simulink library "robot2"
libraries: AtomicLibrary x3, BusImpl x1

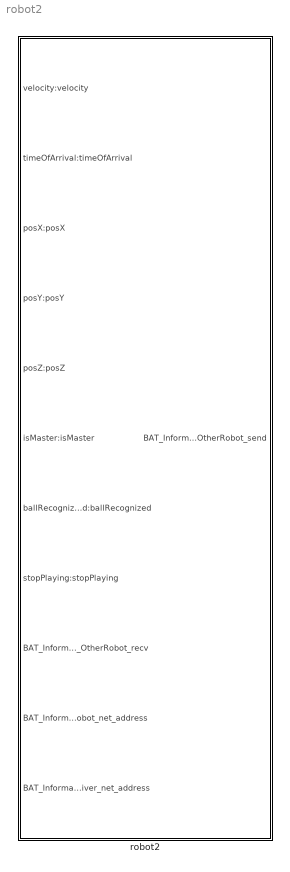
== system robot2 ==
  robot2 : Subsystem  Tag=id=_Sbbd0KYDEeKR7Lwk7UC7tQ

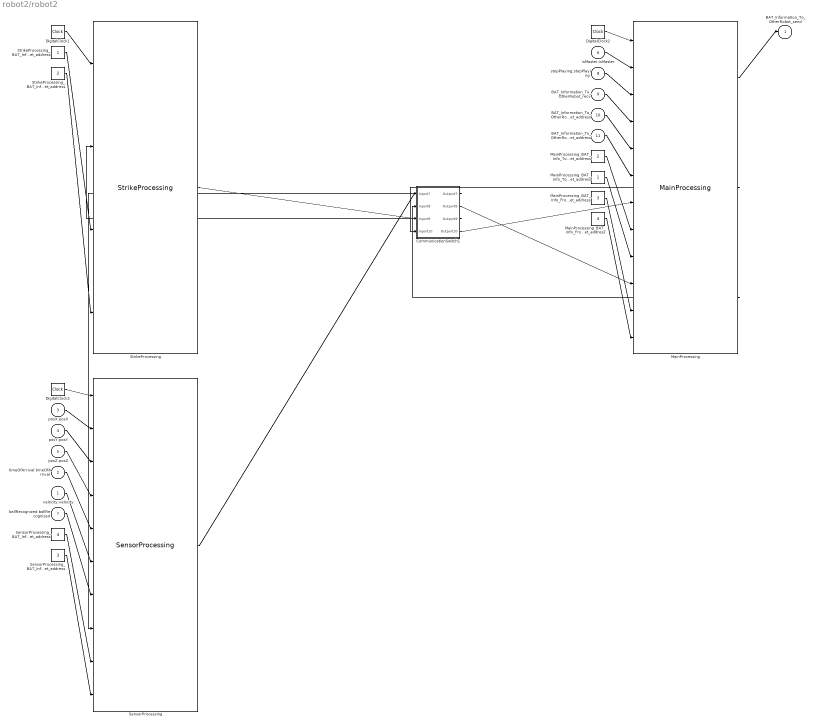
== system robot2/robot2 ==
  velocity:velocity : Inport  Tag=id=_Tii24KYDEeKR7Lwk7UC7tQ  Port=1  DataType=double  OutDataType=fixdt(1, 16)  OutScaling=2^0  OutDataTypeStr=double
  timeOfArrival:timeOfArrival : Inport  Tag=id=_Tiz8oKYDEeKR7Lwk7UC7tQ  Port=2  DataType=double  OutDataType=fixdt(1, 16)  OutScaling=2^0  OutDataTypeStr=double
  posX:posX : Inport  Tag=id=_TjJT0KYDEeKR7Lwk7UC7tQ  Port=3  DataType=double  OutDataType=fixdt(1, 16)  OutScaling=2^0  OutDataTypeStr=double
  posY:posY : Inport  Tag=id=_TjggMKYDEeKR7Lwk7UC7tQ  Port=4  DataType=double  OutDataType=fixdt(1, 16)  OutScaling=2^0  OutDataTypeStr=double
  posZ:posZ : Inport  Tag=id=_TkD50KYDEeKR7Lwk7UC7tQ  Port=5  DataType=double  OutDataType=fixdt(1, 16)  OutScaling=2^0  OutDataTypeStr=double
  isMaster:isMaster : Inport  Tag=id=_TkewkKYDEeKR7Lwk7UC7tQ  Port=6  DataType=boolean  OutDataType=fixdt(1, 16)  OutScaling=2^0  OutDataTypeStr=boolean
  ballRecognized:ballRecognized : Inport  Tag=id=_Tk0u0KYDEeKR7Lwk7UC7tQ  Port=7  DataType=boolean  OutDataType=fixdt(1, 16)  OutScaling=2^0  OutDataTypeStr=boolean
  stopPlaying:stopPlaying : Inport  Tag=id=_TlLUIKYDEeKR7Lwk7UC7tQ  Port=8  DataType=boolean  OutDataType=fixdt(1, 16)  OutScaling=2^0  OutDataTypeStr=boolean
  BAT_Information_To_OtherRobot_recv : Inport  Tag=id=_TmKLkKYDEeKR7Lwk7UC7tQ  Port=9  DataType=auto  OutDataType=fixdt(1, 16)  OutScaling=2^0  UseBusObject=on  OutDataTypeStr=Inherit: auto
      settings: BusObject=PacketBus
  BAT_Information_To_OtherRobot_net_address : Inport  Tag=id=_TmKyoKYDEeKR7Lwk7UC7tQ  Port=10  DataType=uint8  OutDataType=fixdt(1, 16)  OutScaling=2^0  OutDataTypeStr=uint8
  BAT_Information_To_OtherRobot_receiver_net_address : Inport  Tag=id=_TmLZsKYDEeKR7Lwk7UC7tQ  Port=11  DataType=uint8  OutDataType=fixdt(1, 16)  OutScaling=2^0  OutDataTypeStr=uint8
  BAT_Information_To_OtherRobot_send : Outport  Tag=id=_TmKLkaYDEeKR7Lwk7UC7tQ  Port=1  DataType=auto  OutDataType=fixdt(1, 16)  OutScaling=2^0  UseBusObject=on  OutDataTypeStr=Inherit: auto
      settings: BusObject=PacketBus
  CommunicationSwitch1 : Subsystem  Tag=id=_Sbcr8KYDEeKR7Lwk7UC7tQ  LoadFcn=MainBusGenerator
  StrikeProcessing : AtomicLibrary/StrikeProcessing  Tag=id=_Sc3BMKYDEeKR7Lwk7UC7tQ
  DigitalClock1 : DigitalClock  Tag=id=_Sc4PUKYDEeKR7Lwk7UC7tQ  SampleTime=0.0010
  MainProcessing : AtomicLibrary/MainProcessing  Tag=id=_SdIG8KYDEeKR7Lwk7UC7tQ
  DigitalClock2 : DigitalClock  Tag=id=_SdJ8IKYDEeKR7Lwk7UC7tQ  SampleTime=0.0010
  SensorProcessing : AtomicLibrary/SensorProcessing  Tag=id=_SdSfAKYDEeKR7Lwk7UC7tQ
  DigitalClock3 : DigitalClock  Tag=id=_SdTGEKYDEeKR7Lwk7UC7tQ  SampleTime=0.0010
  StrikeProcessing_BAT_Info1_net_address : Constant  Tag=id=_Tc9MQKYDEeKR7Lwk7UC7tQ  Value=1  OutDataTypeMode=uint8  OutDataTypeStr=uint8
  MainProcessing_BAT_Info_ToStrikeProcessing1_net_address : Constant  Tag=id=_TdO5EaYDEeKR7Lwk7UC7tQ  Value=2  OutDataTypeMode=uint8  OutDataTypeStr=uint8
  MainProcessing_BAT_Info_From_SensorProcessing1_net_address : Constant  Tag=id=_TdhM8aYDEeKR7Lwk7UC7tQ  Value=3  OutDataTypeMode=uint8  OutDataTypeStr=uint8
  SensorProcessing_BAT_Info1_net_address : Constant  Tag=id=_Td4ZUaYDEeKR7Lwk7UC7tQ  Value=4  OutDataTypeMode=uint8  OutDataTypeStr=uint8
  SensorProcessing_BAT_Info1_receiver_net_address : Constant  Tag=id=_VS1v0qYDEeKR7Lwk7UC7tQ  Value=3  OutDataTypeMode=uint8  OutDataTypeStr=uint8
  MainProcessing_BAT_Info_From_SensorProcessing1_receiver_net_address : Constant  Tag=id=_VS298KYDEeKR7Lwk7UC7tQ  Value=4  OutDataTypeMode=uint8  OutDataTypeStr=uint8
  StrikeProcessing_BAT_Info1_receiver_net_address : Constant  Tag=id=_VS_g0aYDEeKR7Lwk7UC7tQ  Value=2  OutDataTypeMode=uint8  OutDataTypeStr=uint8
  MainProcessing_BAT_Info_ToStrikeProcessing1_receiver_net_address : Constant  Tag=id=_VTAu8KYDEeKR7Lwk7UC7tQ  Value=1  OutDataTypeMode=uint8  OutDataTypeStr=uint8
  wires:
  DigitalClock1/1 -> StrikeProcessing/1
  DigitalClock2/1 -> MainProcessing/1
  DigitalClock3/1 -> SensorProcessing/1
  StrikeProcessing_BAT_Info1_net_address/1 -> StrikeProcessing/3
  MainProcessing_BAT_Info_ToStrikeProcessing1_net_address/1 -> MainProcessing/8
  MainProcessing_BAT_Info_From_SensorProcessing1_net_address/1 -> MainProcessing/11
  SensorProcessing_BAT_Info1_net_address/1 -> SensorProcessing/9
  SensorProcessing/1 -> CommunicationSwitch1/1(Inport7)
  MainProcessing/3 -> CommunicationSwitch1/2(Inport8)
  CommunicationSwitch1/2(Outport8) -> MainProcessing/10
  CommunicationSwitch1/1(Outport7) -> SensorProcessing/8
  SensorProcessing_BAT_Info1_receiver_net_address/1 -> SensorProcessing/10
  MainProcessing_BAT_Info_From_SensorProcessing1_receiver_net_address/1 -> MainProcessing/12
  StrikeProcessing/1 -> CommunicationSwitch1/3(Inport9)
  MainProcessing/2 -> CommunicationSwitch1/4(Inport10)
  CommunicationSwitch1/4(Outport10) -> MainProcessing/7
  CommunicationSwitch1/3(Outport9) -> StrikeProcessing/2
  StrikeProcessing_BAT_Info1_receiver_net_address/1 -> StrikeProcessing/4
  MainProcessing_BAT_Info_ToStrikeProcessing1_receiver_net_address/1 -> MainProcessing/9
  isMaster:isMaster/1 -> MainProcessing/2
  stopPlaying:stopPlaying/1 -> MainProcessing/3
  ballRecognized:ballRecognized/1 -> SensorProcessing/7
  velocity:velocity/1 -> SensorProcessing/6
  posY:posY/1 -> SensorProcessing/3
  timeOfArrival:timeOfArrival/1 -> SensorProcessing/5
  posX:posX/1 -> SensorProcessing/2
  posZ:posZ/1 -> SensorProcessing/4
  BAT_Information_To_OtherRobot_recv/1 -> MainProcessing/4
  MainProcessing/1 -> BAT_Information_To_OtherRobot_send/1
  BAT_Information_To_OtherRobot_receiver_net_address/1 -> MainProcessing/6
  BAT_Information_To_OtherRobot_net_address/1 -> MainProcessing/5

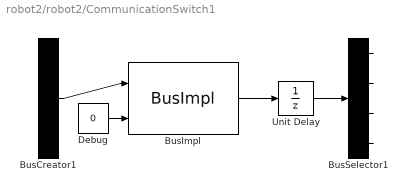
== system robot2/robot2/CommunicationSwitch1 ==
  Inport7 : Inport  Tag=id=_VS1IxKYDEeKR7Lwk7UC7tQ  Port=1  DataType=auto  OutDataType=fixdt(1, 16)  OutScaling=2^0  UseBusObject=on  OutDataTypeStr=Inherit: auto
      settings: BusObject=PacketBus
  Inport8 : Inport  Tag=id=_VS1IxqYDEeKR7Lwk7UC7tQ  Port=2  DataType=auto  OutDataType=fixdt(1, 16)  OutScaling=2^0  UseBusObject=on  OutDataTypeStr=Inherit: auto
      settings: BusObject=PacketBus
  Inport9 : Inport  Tag=id=_VS-5wqYDEeKR7Lwk7UC7tQ  Port=3  DataType=auto  OutDataType=fixdt(1, 16)  OutScaling=2^0  UseBusObject=on  OutDataTypeStr=Inherit: auto
      settings: BusObject=PacketBus
  Inport10 : Inport  Tag=id=_VS-5xKYDEeKR7Lwk7UC7tQ  Port=4  DataType=auto  OutDataType=fixdt(1, 16)  OutScaling=2^0  UseBusObject=on  OutDataTypeStr=Inherit: auto
      settings: BusObject=PacketBus
  Outport7 : Outport  Tag=id=_VS1IxaYDEeKR7Lwk7UC7tQ  Port=1  DataType=auto  OutDataType=fixdt(1, 16)  OutScaling=2^0  UseBusObject=on  OutDataTypeStr=Inherit: auto
      settings: BusObject=PacketBus
  Outport8 : Outport  Tag=id=_VS1Ix6YDEeKR7Lwk7UC7tQ  Port=2  DataType=auto  OutDataType=fixdt(1, 16)  OutScaling=2^0  UseBusObject=on  OutDataTypeStr=Inherit: auto
      settings: BusObject=PacketBus
  Outport9 : Outport  Tag=id=_VS-5w6YDEeKR7Lwk7UC7tQ  Port=3  DataType=auto  OutDataType=fixdt(1, 16)  OutScaling=2^0  UseBusObject=on  OutDataTypeStr=Inherit: auto
      settings: BusObject=PacketBus
  Outport10 : Outport  Tag=id=_VS-5xaYDEeKR7Lwk7UC7tQ  Port=4  DataType=auto  OutDataType=fixdt(1, 16)  OutScaling=2^0  UseBusObject=on  OutDataTypeStr=Inherit: auto
      settings: BusObject=PacketBus
  BusCreator1 : BusCreator  Inputs=4  UseBusObject=on
      settings: BusObject=MainBus
  BusSelector1 : BusSelector  OutputSignals=rc1,rc2,rc3,rc4
  Unit Delay : UnitDelay  SampleTime=-1
  BusImpl : BusImpl/BusImpl
  Debug : Constant  Value=0  OutDataType=fixdt(1, 16)  OutScaling=2^0
  wires:
  BusImpl/1 -> Unit Delay/1
  BusCreator1/1 -> BusImpl/1
  Unit Delay/1 -> BusSelector1/1
  Inport7/1 -> BusCreator1/1  "rc1"
  Inport8/1 -> BusCreator1/2  "rc2"
  Inport9/1 -> BusCreator1/3  "rc3"
  Inport10/1 -> BusCreator1/4  "rc4"
  BusSelector1/1 -> Outport7/1
  BusSelector1/2 -> Outport8/1
  BusSelector1/3 -> Outport9/1
  BusSelector1/4 -> Outport10/1
  Debug/1 -> BusImpl/2
